simulink subsystem "StateCovarianceInit"  (R2021a)
settings: Solver=VariableStepAuto  StartTime=0.0  StopTime=10.0  RelTol=1e-3
undefined symbols (not defined in the file): imu1, imu2, imu3, imu4, magnitude
libraries: dspmtrx3 x1
settings Model: Creator=Laura  LastModifiedBy=Laura

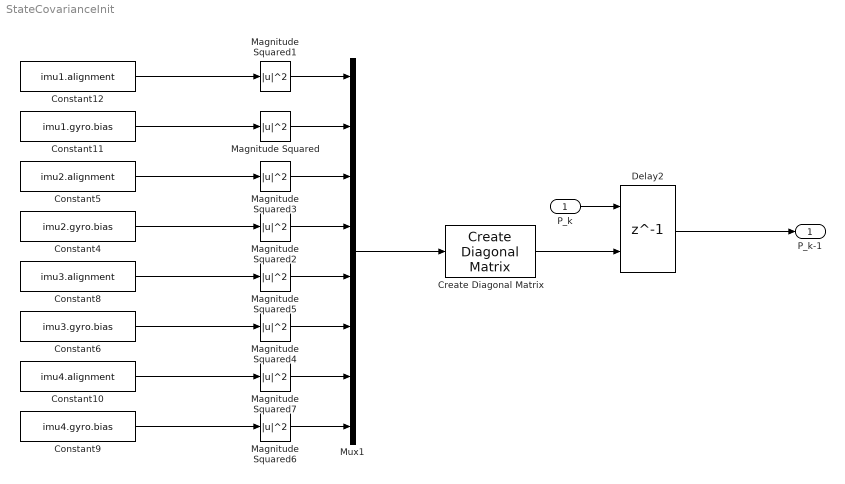
== system StateCovarianceInit ==
  P_k : Inport
  Constant10 : Constant  Value=imu4.alignment
  Constant11 : Constant  Value=imu1.gyro.bias
  Constant12 : Constant  Value=imu1.alignment
  Constant4 : Constant  Value=imu2.gyro.bias
  Constant5 : Constant  Value=imu2.alignment
  Constant6 : Constant  Value=imu3.gyro.bias
  Constant8 : Constant  Value=imu3.alignment
  Constant9 : Constant  Value=imu4.gyro.bias
  Create Diagonal Matrix : dspmtrx3/Create Diagonal Matrix
      settings: SourceProductBaseCode=DS
  Delay2 : Delay  DelayLength=1  InitialConditionSource=Input port
      settings: InputPortMap=u0,p4
  Magnitude Squared{,1..7} (8 alike) : Math  Operator=magnitude^2  SaturateOnIntegerOverflow=on
  Mux1 : Mux  Inputs=8
  P_k-1 : Outport
  wires:
  Mux1/1 -> Create Diagonal Matrix/1
  P_k/1 -> Delay2/1
  Create Diagonal Matrix/1 -> Delay2/2
  Delay2/1 -> P_k-1/1
  Constant9/1 -> Magnitude Squared6/1
  Magnitude Squared2/1 -> Mux1/4
  Constant12/1 -> Magnitude Squared1/1
  Magnitude Squared4/1 -> Mux1/6
  Magnitude Squared1/1 -> Mux1/1
  Constant8/1 -> Magnitude Squared5/1
  Magnitude Squared7/1 -> Mux1/7
  Magnitude Squared3/1 -> Mux1/3
  Constant11/1 -> Magnitude Squared/1
  Constant4/1 -> Magnitude Squared2/1
  Constant10/1 -> Magnitude Squared7/1
  Magnitude Squared/1 -> Mux1/2
  Constant5/1 -> Magnitude Squared3/1
  Magnitude Squared5/1 -> Mux1/5
  Magnitude Squared6/1 -> Mux1/8
  Constant6/1 -> Magnitude Squared4/1
